simulink model "CruiseControl"  (R2017a)
settings: Solver=VariableStepAuto  StartTime=0.0  StopTime=600  RelTol=1e-3
settings Model: Creator=giulio.giorgione  LastModifiedBy=giulio.giorgione

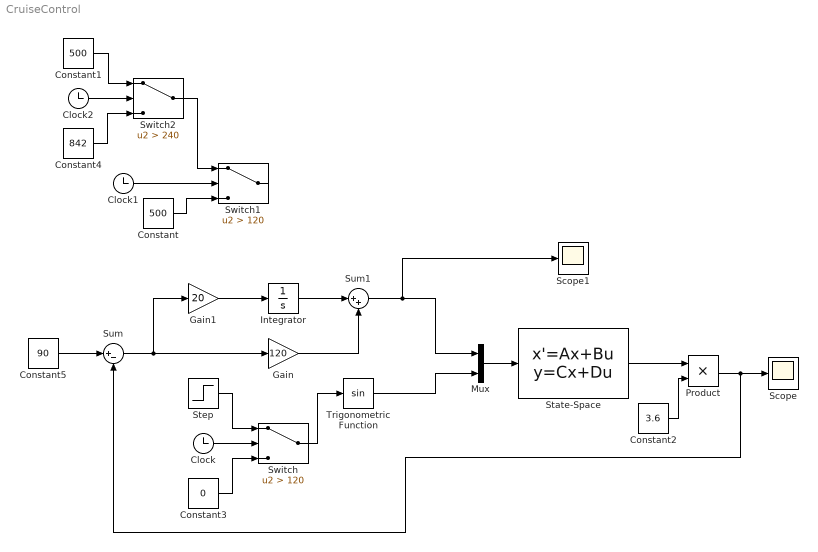
== system CruiseControl ==
  Clock : Clock
  Clock1 : Clock
  Clock2 : Clock
  Constant : Constant  Value=500
  Constant1 : Constant  Value=500
  Constant2 : Constant  Value=3.6
  Constant3 : Constant  Value=0
  Constant4 : Constant  Value=842
  Constant5 : Constant  Value=90
  Gain : Gain  Gain=120
  Gain1 : Gain  Gain=20
  Integrator : Integrator
  Mux : Mux  Inputs=2
  Product : Product
  Scope : Scope
  Scope1 : Scope
  State-Space : StateSpace  A=-0.02  B=[0.001,-9.8]  D=[0, 0]  X0=90/3.6
  Step : Step  Time=240  Before=pi/2*2/90  After=0  SampleTime=120
  Sum : Sum  Inputs=|+-
  Sum1 : Sum  Inputs=|++
  Switch : Switch  Criteria=u2 > Threshold  Threshold=120
  Switch1 : Switch  Criteria=u2 > Threshold  Threshold=120
  Switch2 : Switch  Criteria=u2 > Threshold  Threshold=240
  Trigonometric Function : Trigonometry
  wires:
  State-Space/1 -> Product/1
  Constant/1 -> Switch1/3
  Step/1 -> Switch/1
  Mux/1 -> State-Space/1
  Constant2/1 -> Product/2
  Product/1 -> Sum/2, Scope/1
  Trigonometric Function/1 -> Mux/2
  Clock/1 -> Switch/2
  Constant3/1 -> Switch/3
  Switch/1 -> Trigonometric Function/1
  Constant5/1 -> Sum/1
  Clock1/1 -> Switch1/2
  Switch2/1 -> Switch1/1
  Constant4/1 -> Switch2/3
  Constant1/1 -> Switch2/1
  Clock2/1 -> Switch2/2
  Sum/1 -> Gain1/1, Gain/1
  Gain/1 -> Sum1/2
  Integrator/1 -> Sum1/1
  Sum1/1 -> Scope1/1, Mux/1
  Gain1/1 -> Integrator/1
